simulink model "FCS"  (Simulink 9.1)
settings: Solver=VariableStepAuto  StartTime=0.0  StopTime=10.0  RelTol=1e-3
values from neighbouring files (symbols this model uses):
  Controller =     [data_set.mat]
  Estimator =     [data_set.mat]
  g = 9.81    [data_set.mat]
  init =     [data_set.mat]
  Sensors =     [data_set.mat]
  Ts = 0.005    [data_set.mat]
  Vehicle =     [data_set.mat]
undefined symbols (not defined in the file or in its folder): DiscIntNeverNeededParam, Discrete, Time
libraries: F_Line_block x470, simulink x33, ctrlSharedLib x3, sharedtransform x3, sharedutil x1
(part 1 of 3)
settings Model: LogicAnalyzerSignalOrdering=db974c0d-bb14-49c7-94ac-ee659e6fa1a8,d1d32620-0112-4d85-a8d5-fcd62d13050a  Creator=dongw  LastModifiedBy=dongw
settings DataIOCC: SaveFormat=Dataset
settings OptimizationCC: LifeSpan=auto
settings DebuggingCC: UnderspecifiedInitializationDetection=Simplified  MergeDetectMultiDrivingBlocksExec=error  SFUnexpectedBacktrackingDiag=error  SFNoUnconditionalDefaultTransitionDiag=error  SFExecutionAtInitializationDiag=warning
settings HardwareCC: ProdBitPerPointer=64  ProdBitPerSizeT=64  ProdBitPerPtrDiffT=64  ProdLargestAtomicFloat=Float  ProdIntDivRoundTo=Zero  ProdEndianess=LittleEndian  ProdWordSize=64  ProdHWDeviceType=Intel->x86-64 (Windows64)
settings ModelReferenceCC: PropagateSignalLabelsOutOfModel=on
settings CodeAppCC: StateflowObjectComments=off
settings GRTTargetCC: TargetLangStandard=C99 (ISO)  CombineOutputUpdateFcns=on  GRTInterface=off
settings ConfigComp: CovMetricSettings=dwe  CovHtmlReporting=off  CovSaveCumulativeToWorkspaceVar=off  CovSaveSingleToWorkspaceVar=off  CovExternalEMLEnable=on

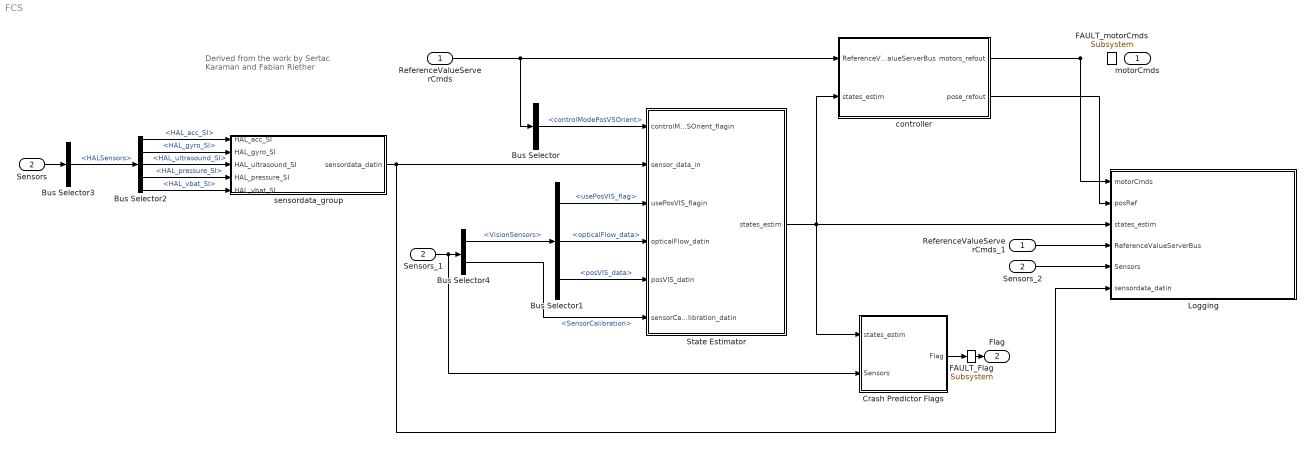
== system FCS ==
  note: Derived from the work by Sertac
      | Karaman and Fabian Riether
  ReferenceValueServerCmds : Inport  OutDataTypeStr=Bus: CommandBus
  Sensors : Inport  Port=2  OutDataTypeStr=Bus: SensorsBus  BusOutputAsStruct=on
  Bus Selector : BusSelector  OutputSignals=controlModePosVSOrient
  Bus Selector1 : BusSelector  OutputSignals=usePosVIS_flag,opticalFlow_data,posVIS_data
  Bus Selector2 : BusSelector  OutputSignals=HAL_acc_SI,HAL_gyro_SI,HAL_ultrasound_SI,HAL_pressure_SI,HAL_vbat_SI
  Bus Selector3 : BusSelector  OutputSignals=HALSensors
  Bus Selector4 : BusSelector  OutputSignals=VisionSensors,SensorCalibration
  Crash Predictor Flags : Subsystem
  Logging : Subsystem  TreatAsAtomicUnit=on
      settings: RTWFcnNameOpts=Use subsystem name
  ReferenceValueServerCmds_1 : InportShadow  OutDataTypeStr=Bus: CommandBus
  Sensors_1 : InportShadow  Port=2  OutDataTypeStr=Bus: SensorsBus  BusOutputAsStruct=on
  Sensors_2 : InportShadow  Port=2  OutDataTypeStr=Bus: SensorsBus  BusOutputAsStruct=on
  State Estimator : Subsystem
  controller : Subsystem
  sensordata_group : Subsystem
  motorCmds : Outport
  FAULT_motorCmds : F_Line_block/Subsystem
  Flag : Outport  Port=2
  FAULT_Flag : F_Line_block/Subsystem
  wires:
  sensordata_group/1(sensordata_datin) -> State Estimator/2(sensor_data_in), Logging/6(sensordata_datin)
  Bus Selector1/2 -> State Estimator/4(opticalFlow_datin)  "<opticalFlow_data>"
  Sensors_1/1 -> Crash Predictor Flags/2(Sensors), Bus Selector4/1
  Bus Selector2/3 -> sensordata_group/3(HAL_ultrasound_SI)  "<HAL_ultrasound_SI>"
  Bus Selector/1 -> State Estimator/1(controlModePosVSOrient_flagin)  "<controlModePosVSOrient>"
  Sensors/1 -> Bus Selector3/1
  Sensors_2/1 -> Logging/5(Sensors)
  Bus Selector2/2 -> sensordata_group/2(HAL_gyro_SI)  "<HAL_gyro_SI>"
  Bus Selector4/2 -> State Estimator/6(sensorCalibration_datin)  "<SensorCalibration>"
  Crash Predictor Flags/1(Flag) -> FAULT_Flag/1
  ?FAULT_Sum4_		DstPort			1/1 -> ?Sum4/dstport			1
  ?FAULT_Mux2_3/1 -> ?Mux2/3
  ?FAULT_pitch_roll_cmd/1 -> ?pitch_roll_cmd/1
  ?FAULT_Out Bus Element7/1 -> ?Out Bus Element7/1
  ?FAULT_Delay1/1 -> ?Delay1/1
  ?FAULT_Demux3/1 -> ?Demux3/1
  FAULT_Flag/1 -> Flag/1
  controller/1(motors_refout) -> ?FAULT_motorCmds_	DstPort			1/1, Logging/1(motorCmds)
  ?FAULT_motorCmds_	DstPort			1/1 -> motorCmds/dstport			1
  ?FAULT_Mux2_3/1 -> ?Mux2/3
  Bus Selector1/1 -> State Estimator/3(usePosVIS_flagin)  "<usePosVIS_flag>"
  Bus Selector1/3 -> State Estimator/5(posVIS_datin)  "<posVIS_data>"
  Bus Selector2/1 -> sensordata_group/1(HAL_acc_SI)  "<HAL_acc_SI>"
  controller/2(pose_refout) -> Logging/2(posRef)
  ReferenceValueServerCmds_1/1 -> Logging/4(ReferenceValueServerBus)
  Bus Selector4/1 -> Bus Selector1/1  "<VisionSensors>"
  State Estimator/1(states_estim) -> controller/2(states_estim), Crash Predictor Flags/1(states_estim), Logging/3(states_estim)
  Bus Selector2/5 -> sensordata_group/5(HAL_vbat_SI)  "<HAL_vbat_SI>"
  Bus Selector2/4 -> sensordata_group/4(HAL_pressure_SI)  "<HAL_pressure_SI>"
  Bus Selector3/1 -> Bus Selector2/1  "<HALSensors>"
  ReferenceValueServerCmds/1 -> controller/1(ReferenceValueServerBus), Bus Selector/1

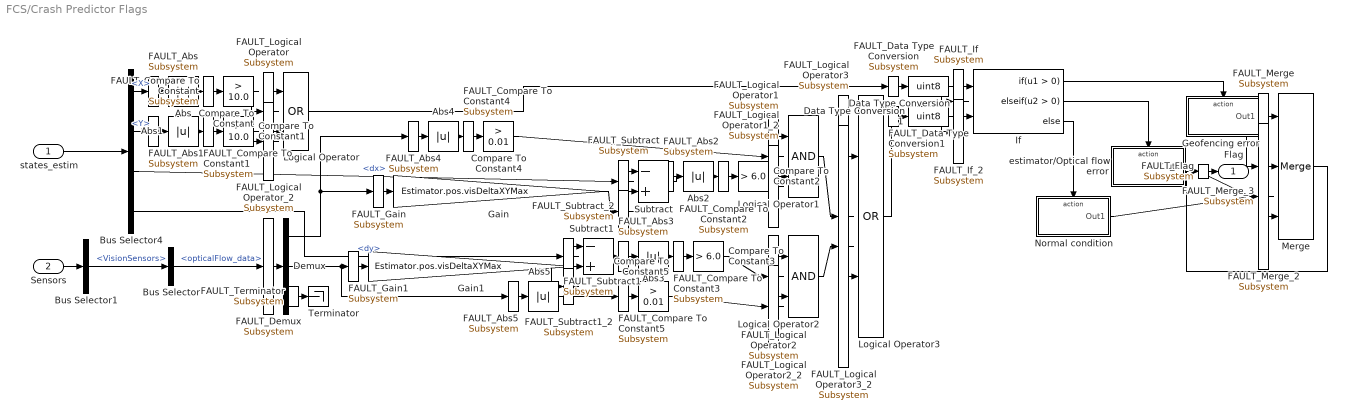
== system FCS/Crash Predictor Flags ==
  states_estim : Inport
  Sensors : Inport  Port=2
  Abs{,1..5} (6 alike) : Abs
  FAULT_Abs{,1..5} (6 alike) : F_Line_block/Subsystem
  Bus Selector : BusSelector  OutputSignals=opticalFlow_data
  Bus Selector1 : BusSelector  OutputSignals=VisionSensors
  Bus Selector4 : BusSelector  OutputSignals=X,Y,dx,dy
  Compare To Constant : simulink/Logic and Bit Operations/Compare To Constant  relop=>  const=10.0  OutDataTypeStr=boolean
  FAULT_Compare To Constant{,1..5} (6 alike) : F_Line_block/Subsystem
  Compare To Constant1 : simulink/Logic and Bit Operations/Compare To Constant  relop=>  const=10.0  OutDataTypeStr=boolean
  Compare To Constant2 : simulink/Logic and Bit Operations/Compare To Constant  relop=>  const=6.0  OutDataTypeStr=boolean
  Compare To Constant3 : simulink/Logic and Bit Operations/Compare To Constant  relop=>  const=6.0  OutDataTypeStr=boolean
  Compare To Constant4 : simulink/Logic and Bit Operations/Compare To Constant  relop=>  const=0.01  OutDataTypeStr=boolean
  Compare To Constant5 : simulink/Logic and Bit Operations/Compare To Constant  relop=>  const=0.01  OutDataTypeStr=boolean
  Data Type Conversion : DataTypeConversion  OutDataTypeStr=uint8  RndMeth=Nearest
  FAULT_Data Type Conversion : F_Line_block/Subsystem
  Data Type Conversion1 : DataTypeConversion  OutDataTypeStr=uint8  RndMeth=Nearest
  FAULT_Data Type Conversion1 : F_Line_block/Subsystem
  Demux : Demux  Outputs=3
  FAULT_Demux : F_Line_block/Subsystem
  Gain : Gain  Gain=Estimator.pos.visDeltaXYMax
  FAULT_Gain : F_Line_block/Subsystem
  Gain1 : Gain  Gain=Estimator.pos.visDeltaXYMax
  FAULT_Gain1 : F_Line_block/Subsystem
  Geofencing error : Subsystem  TreatAsAtomicUnit=on
  If : If  NumInputs=2  ElseIfExpressions=u2 > 0
  FAULT_If : F_Line_block/Subsystem
  FAULT_If_2 : F_Line_block/Subsystem
  Logical Operator : Logic  Operator=OR  AllPortsSameDT=off
  FAULT_Logical Operator{,1..3} (4 alike) : F_Line_block/Subsystem
  FAULT_Logical Operator_2 : F_Line_block/Subsystem
  Logical Operator1 : Logic  AllPortsSameDT=off  OutDataTypeStr=boolean
  FAULT_Logical Operator1_2 : F_Line_block/Subsystem
  Logical Operator2 : Logic  AllPortsSameDT=off  OutDataTypeStr=boolean
  FAULT_Logical Operator2_2 : F_Line_block/Subsystem
  Logical Operator3 : Logic  Operator=OR  AllPortsSameDT=off
  FAULT_Logical Operator3_2 : F_Line_block/Subsystem
  Merge : Merge  Inputs=3  InitialOutput=0
  FAULT_Merge : F_Line_block/Subsystem
  FAULT_Merge_2 : F_Line_block/Subsystem
  FAULT_Merge_3 : F_Line_block/Subsystem
  Normal condition : Subsystem  TreatAsAtomicUnit=on
  Subtract : Sum  Inputs=-+
  FAULT_Subtract : F_Line_block/Subsystem
  FAULT_Subtract_2 : F_Line_block/Subsystem
  Subtract1 : Sum  Inputs=-+
  FAULT_Subtract1 : F_Line_block/Subsystem
  FAULT_Subtract1_2 : F_Line_block/Subsystem
  Terminator : Terminator
  FAULT_Terminator : F_Line_block/Subsystem
  estimator/Optical flow error : Subsystem  TreatAsAtomicUnit=on
  Flag : Outport
  FAULT_Flag : F_Line_block/Subsystem
  wires:
  Bus Selector4/1 -> FAULT_Abs/1  "<X>"
  FAULT_Abs/1 -> Abs/1
  states_estim/1 -> Bus Selector4/1
  Bus Selector4/2 -> FAULT_Abs1/1  "<Y>"
  FAULT_Abs1/1 -> Abs1/1
  Compare To Constant/1 -> FAULT_Logical Operator/1
  FAULT_Logical Operator/1 -> Logical Operator/1
  Compare To Constant1/1 -> FAULT_Logical Operator_2/1
  FAULT_Logical Operator_2/1 -> Logical Operator/2
  Abs/1 -> FAULT_Compare To Constant/1
  FAULT_Compare To Constant/1 -> Compare To Constant/1
  Abs1/1 -> FAULT_Compare To Constant1/1
  FAULT_Compare To Constant1/1 -> Compare To Constant1/1
  Logical Operator/1 -> FAULT_Data Type Conversion/1
  FAULT_Data Type Conversion/1 -> Data Type Conversion/1
  Bus Selector/1 -> FAULT_Demux/1  "<opticalFlow_data>"
  FAULT_Demux/1 -> Demux/1
  Demux/1 -> FAULT_Abs4/1, FAULT_Gain/1
  FAULT_Abs4/1 -> Abs4/1
  FAULT_Gain/1 -> Gain/1
  Demux/2 -> FAULT_Gain1/1, FAULT_Abs5/1
  FAULT_Gain1/1 -> Gain1/1
  FAULT_Abs5/1 -> Abs5/1
  Bus Selector4/3 -> FAULT_Subtract/1  "<dx>"
  FAULT_Subtract/1 -> Subtract/1
  Subtract/1 -> FAULT_Abs2/1
  FAULT_Abs2/1 -> Abs2/1
  Subtract1/1 -> FAULT_Abs3/1
  FAULT_Abs3/1 -> Abs3/1
  Abs2/1 -> FAULT_Compare To Constant2/1
  FAULT_Compare To Constant2/1 -> Compare To Constant2/1
  Abs3/1 -> FAULT_Compare To Constant3/1
  FAULT_Compare To Constant3/1 -> Compare To Constant3/1
  Compare To Constant5/1 -> FAULT_Logical Operator2_2/1
  FAULT_Logical Operator2_2/1 -> Logical Operator2/2
  Abs4/1 -> FAULT_Compare To Constant4/1
  FAULT_Compare To Constant4/1 -> Compare To Constant4/1
  Abs5/1 -> FAULT_Compare To Constant5/1
  FAULT_Compare To Constant5/1 -> Compare To Constant5/1
  Compare To Constant3/1 -> FAULT_Logical Operator2/1
  FAULT_Logical Operator2/1 -> Logical Operator2/1
  Logical Operator1/1 -> FAULT_Logical Operator3/1
  FAULT_Logical Operator3/1 -> Logical Operator3/1
  Logical Operator2/1 -> FAULT_Logical Operator3_2/1
  FAULT_Logical Operator3_2/1 -> Logical Operator3/2
  Logical Operator3/1 -> FAULT_Data Type Conversion1/1
  FAULT_Data Type Conversion1/1 -> Data Type Conversion1/1
  Demux/3 -> FAULT_Terminator/1
  FAULT_Terminator/1 -> Terminator/1
  Gain/1 -> FAULT_Subtract_2/1
  FAULT_Subtract_2/1 -> Subtract/2
  Bus Selector4/4 -> FAULT_Subtract1/1  "<dy>"
  FAULT_Subtract1/1 -> Subtract1/1
  Gain1/1 -> FAULT_Subtract1_2/1
  FAULT_Subtract1_2/1 -> Subtract1/2
  Compare To Constant4/1 -> FAULT_Logical Operator1/1
  FAULT_Logical Operator1/1 -> Logical Operator1/1
  Compare To Constant2/1 -> FAULT_Logical Operator1_2/1
  FAULT_Logical Operator1_2/1 -> Logical Operator1/2
  Sensors/1 -> Bus Selector1/1
  Bus Selector1/1 -> Bus Selector/1  "<VisionSensors>"
  Merge/1 -> FAULT_Flag/1
  FAULT_Flag/1 -> Flag/1
  If/1 -> Geofencing error/Action
  If/2 -> estimator/Optical flow error/Action
  If/3 -> Normal condition/Action
  Geofencing error/1(Out1) -> FAULT_Merge/1
  FAULT_Merge/1 -> Merge/1
  estimator/Optical flow error/1(Out1) -> FAULT_Merge_2/1
  FAULT_Merge_2/1 -> Merge/2
  Normal condition/1(Out1) -> FAULT_Merge_3/1
  FAULT_Merge_3/1 -> Merge/3
  Data Type Conversion/1 -> FAULT_If/1
  FAULT_If/1 -> If/1
  Data Type Conversion1/1 -> FAULT_If_2/1
  FAULT_If_2/1 -> If/2

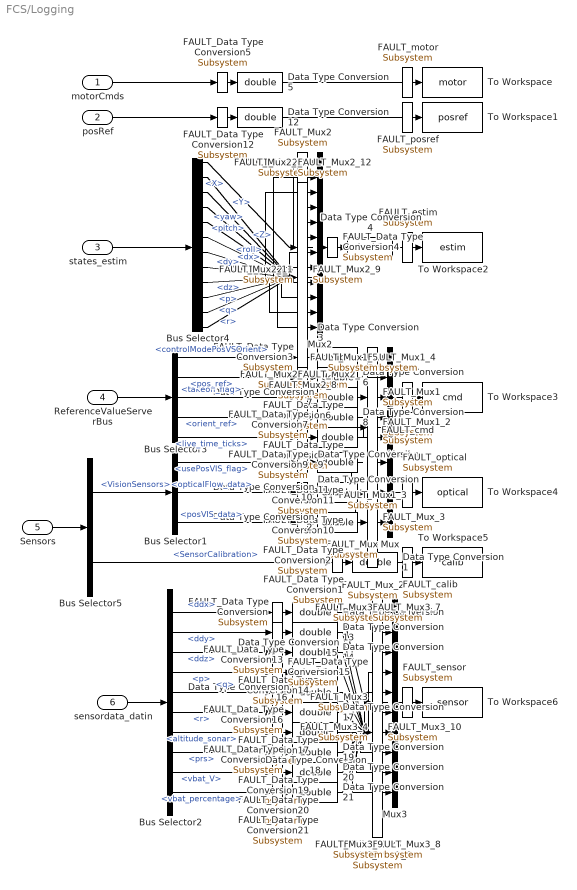
== system FCS/Logging ==
  motorCmds : Inport
  posRef : Inport  Port=2
  states_estim : Inport  Port=3  OutDataTypeStr=Bus: statesEstim_t  BusOutputAsStruct=on
  ReferenceValueServerBus : Inport  Port=4  OutDataTypeStr=Bus: CommandBus  BusOutputAsStruct=on
  Sensors : Inport  Port=5  OutDataTypeStr=Bus: SensorsBus
  sensordata_datin : Inport  Port=6  OutDataTypeStr=Bus: sensordata_t
  Bus Selector1 : BusSelector  OutputSignals=usePosVIS_flag,opticalFlow_data,posVIS_data
  Bus Selector2 : BusSelector  OutputSignals=ddx,ddy,ddz,p,q,r,altitude_sonar,prs,vbat_V,vbat_percentage
  Bus Selector3 : BusSelector  OutputSignals=controlModePosVSOrient,pos_ref,takeoff_flag,orient_ref,live_time_ticks
  Bus Selector4 : BusSelector  OutputSignals=X,Y,Z,yaw,pitch,roll,dx,dy,dz,p,q,r
  Bus Selector5 : BusSelector  OutputSignals=VisionSensors,SensorCalibration
  Data Type Conversion{,1..21} (22 alike) : DataTypeConversion  OutDataTypeStr=double
  FAULT_Data Type Conversion{,1..21} (22 alike) : F_Line_block/Subsystem
  Mux : Mux  Inputs=3
  FAULT_Mux{,1..3} (4 alike) : F_Line_block/Subsystem
  FAULT_Mux_2 : F_Line_block/Subsystem
  FAULT_Mux_3 : F_Line_block/Subsystem
  Mux1 : Mux  Inputs=5
  FAULT_Mux1_{2..5} (4 alike) : F_Line_block/Subsystem
  Mux2 : Mux  Inputs=12
  FAULT_Mux2_{2..12} (11 alike) : F_Line_block/Subsystem
  Mux3 : Mux  Inputs=10
  FAULT_Mux3_{2..10} (9 alike) : F_Line_block/Subsystem
  To Workspace : ToWorkspace  VariableName=motor  SaveFormat=Structure With Time  SampleTime=-1
  FAULT_motor : F_Line_block/Subsystem
  To Workspace1 : ToWorkspace  VariableName=posref  SaveFormat=Structure With Time  SampleTime=-1
  FAULT_posref : F_Line_block/Subsystem
  To Workspace2 : ToWorkspace  VariableName=estim  SaveFormat=Structure With Time  SampleTime=-1
  FAULT_estim : F_Line_block/Subsystem
  To Workspace3 : ToWorkspace  VariableName=cmd  SaveFormat=Structure With Time  SampleTime=-1
  FAULT_cmd : F_Line_block/Subsystem
  To Workspace4 : ToWorkspace  VariableName=optical  SaveFormat=Structure With Time  SampleTime=-1
  FAULT_optical : F_Line_block/Subsystem
  To Workspace5 : ToWorkspace  VariableName=calib  SaveFormat=Structure With Time  SampleTime=-1
  FAULT_calib : F_Line_block/Subsystem
  To Workspace6 : ToWorkspace  VariableName=sensor  SaveFormat=Structure With Time  SampleTime=-1
  FAULT_sensor : F_Line_block/Subsystem
  wires:
  Bus Selector3/1 -> FAULT_Data Type Conversion3/1  "<controlModePosVSOrient>"
  FAULT_Data Type Conversion3/1 -> Data Type Conversion3/1
  Bus Selector3/3 -> FAULT_Data Type Conversion7/1  "<takeoff_flag>"
  FAULT_Data Type Conversion7/1 -> Data Type Conversion7/1
  Bus Selector3/4 -> FAULT_Data Type Conversion8/1  "<orient_ref>"
  FAULT_Data Type Conversion8/1 -> Data Type Conversion8/1
  Bus Selector3/5 -> FAULT_Data Type Conversion9/1  "<live_time_ticks>"
  FAULT_Data Type Conversion9/1 -> Data Type Conversion9/1
  ReferenceValueServerBus/1 -> Bus Selector3/1
  Bus Selector3/2 -> FAULT_Data Type Conversion6/1  "<pos_ref>"
  FAULT_Data Type Conversion6/1 -> Data Type Conversion6/1
  sensordata_datin/1 -> Bus Selector2/1
  Bus Selector2/1 -> FAULT_Data Type Conversion/1  "<ddx>"
  FAULT_Data Type Conversion/1 -> Data Type Conversion/1
  Sensors/1 -> Bus Selector5/1
  Bus Selector1/1 -> FAULT_Data Type Conversion11/1  "<usePosVIS_flag>"
  FAULT_Data Type Conversion11/1 -> Data Type Conversion11/1
  Bus Selector1/2 -> FAULT_Data Type Conversion10/1  "<opticalFlow_data>"
  FAULT_Data Type Conversion10/1 -> Data Type Conversion10/1
  Bus Selector1/3 -> FAULT_Data Type Conversion2/1  "<posVIS_data>"
  FAULT_Data Type Conversion2/1 -> Data Type Conversion2/1
  Data Type Conversion1/1 -> To Workspace5/1
  Bus Selector5/2 -> FAULT_Data Type Conversion1/1  "<SensorCalibration>"
  FAULT_Data Type Conversion1/1 -> Data Type Conversion1/1
  Mux/1 -> To Workspace4/1
  Data Type Conversion4/1 -> To Workspace2/1
  motorCmds/1 -> FAULT_Data Type Conversion5/1
  FAULT_Data Type Conversion5/1 -> Data Type Conversion5/1
  Data Type Conversion5/1 -> To Workspace/1
  Mux1/1 -> To Workspace3/1
  states_estim/1 -> Bus Selector4/1
  Mux2/1 -> FAULT_Data Type Conversion4/1
  FAULT_Data Type Conversion4/1 -> Data Type Conversion4/1
  Bus Selector4/4 -> FAULT_Mux2_4/1  "<yaw>"
  FAULT_Mux2_4/1 -> Mux2/4
  Bus Selector4/6 -> FAULT_Mux2_6/1  "<roll>"
  FAULT_Mux2_6/1 -> Mux2/6
  Bus Selector4/5 -> FAULT_Mux2_5/1  "<pitch>"
  FAULT_Mux2_5/1 -> Mux2/5
  Bus Selector4/9 -> FAULT_Mux2_9/1  "<dz>"
  FAULT_Mux2_9/1 -> Mux2/9
  Bus Selector4/7 -> FAULT_Mux2_7/1  "<dx>"
  FAULT_Mux2_7/1 -> Mux2/7
  Bus Selector4/8 -> FAULT_Mux2_8/1  "<dy>"
  FAULT_Mux2_8/1 -> Mux2/8
  Bus Selector4/10 -> FAULT_Mux2_10/1  "<p>"
  FAULT_Mux2_10/1 -> Mux2/10
  Bus Selector4/12 -> FAULT_Mux2_12/1  "<r>"
  FAULT_Mux2_12/1 -> Mux2/12
  Bus Selector4/2 -> FAULT_Mux2_2/1  "<Y>"
  FAULT_Mux2_2/1 -> Mux2/2
  Bus Selector4/11 -> FAULT_Mux2_11/1  "<q>"
  FAULT_Mux2_11/1 -> Mux2/11
  Bus Selector4/3 -> FAULT_Mux2_3/1  "<Z>"
  FAULT_Mux2_3/1 -> Mux2/3
  Bus Selector4/1 -> FAULT_Mux2/1  "<X>"
  FAULT_Mux2/1 -> Mux2/1
  Data Type Conversion3/1 -> FAULT_Mux1/1
  FAULT_Mux1/1 -> Mux1/1
  Data Type Conversion6/1 -> FAULT_Mux1_2/1
  FAULT_Mux1_2/1 -> Mux1/2
  Data Type Conversion7/1 -> FAULT_Mux1_3/1
  FAULT_Mux1_3/1 -> Mux1/3
  Data Type Conversion8/1 -> FAULT_Mux1_4/1
  FAULT_Mux1_4/1 -> Mux1/4
  Data Type Conversion9/1 -> FAULT_Mux1_5/1
  FAULT_Mux1_5/1 -> Mux1/5
  Data Type Conversion2/1 -> FAULT_Mux_3/1
  FAULT_Mux_3/1 -> Mux/3
  Data Type Conversion10/1 -> FAULT_Mux_2/1
  FAULT_Mux_2/1 -> Mux/2
  Data Type Conversion11/1 -> FAULT_Mux/1
  FAULT_Mux/1 -> Mux/1
  posRef/1 -> FAULT_Data Type Conversion12/1
  FAULT_Data Type Conversion12/1 -> Data Type Conversion12/1
  Data Type Conversion12/1 -> To Workspace1/1
  Bus Selector2/2 -> FAULT_Data Type Conversion13/1  "<ddy>"
  FAULT_Data Type Conversion13/1 -> Data Type Conversion13/1
  Bus Selector2/3 -> FAULT_Data Type Conversion14/1  "<ddz>"
  FAULT_Data Type Conversion14/1 -> Data Type Conversion14/1
  Bus Selector2/4 -> FAULT_Data Type Conversion15/1  "<p>"
  FAULT_Data Type Conversion15/1 -> Data Type Conversion15/1
  Bus Selector2/5 -> FAULT_Data Type Conversion16/1  "<q>"
  FAULT_Data Type Conversion16/1 -> Data Type Conversion16/1
  Bus Selector2/6 -> FAULT_Data Type Conversion17/1  "<r>"
  FAULT_Data Type Conversion17/1 -> Data Type Conversion17/1
  Bus Selector2/7 -> FAULT_Data Type Conversion18/1  "<altitude_sonar>"
  FAULT_Data Type Conversion18/1 -> Data Type Conversion18/1
  Bus Selector2/8 -> FAULT_Data Type Conversion19/1  "<prs>"
  FAULT_Data Type Conversion19/1 -> Data Type Conversion19/1
  Bus Selector2/9 -> FAULT_Data Type Conversion20/1  "<vbat_V>"
  FAULT_Data Type Conversion20/1 -> Data Type Conversion20/1
  Bus Selector2/10 -> FAULT_Data Type Conversion21/1  "<vbat_percentage>"
  FAULT_Data Type Conversion21/1 -> Data Type Conversion21/1
  Data Type Conversion/1 -> FAULT_Mux3/1
  FAULT_Mux3/1 -> Mux3/1
  Data Type Conversion13/1 -> FAULT_Mux3_2/1
  FAULT_Mux3_2/1 -> Mux3/2
  Data Type Conversion14/1 -> FAULT_Mux3_3/1
  FAULT_Mux3_3/1 -> Mux3/3
  Data Type Conversion15/1 -> FAULT_Mux3_4/1
  FAULT_Mux3_4/1 -> Mux3/4
  Data Type Conversion16/1 -> FAULT_Mux3_5/1
  FAULT_Mux3_5/1 -> Mux3/5
  Data Type Conversion17/1 -> FAULT_Mux3_6/1
  FAULT_Mux3_6/1 -> Mux3/6
  Data Type Conversion18/1 -> FAULT_Mux3_7/1
  FAULT_Mux3_7/1 -> Mux3/7
  Data Type Conversion19/1 -> FAULT_Mux3_8/1
  FAULT_Mux3_8/1 -> Mux3/8
  Data Type Conversion20/1 -> FAULT_Mux3_9/1
  FAULT_Mux3_9/1 -> Mux3/9
  Data Type Conversion21/1 -> FAULT_Mux3_10/1
  FAULT_Mux3_10/1 -> Mux3/10
  Mux3/1 -> To Workspace6/1
  Bus Selector5/1 -> Bus Selector1/1  "<VisionSensors>"

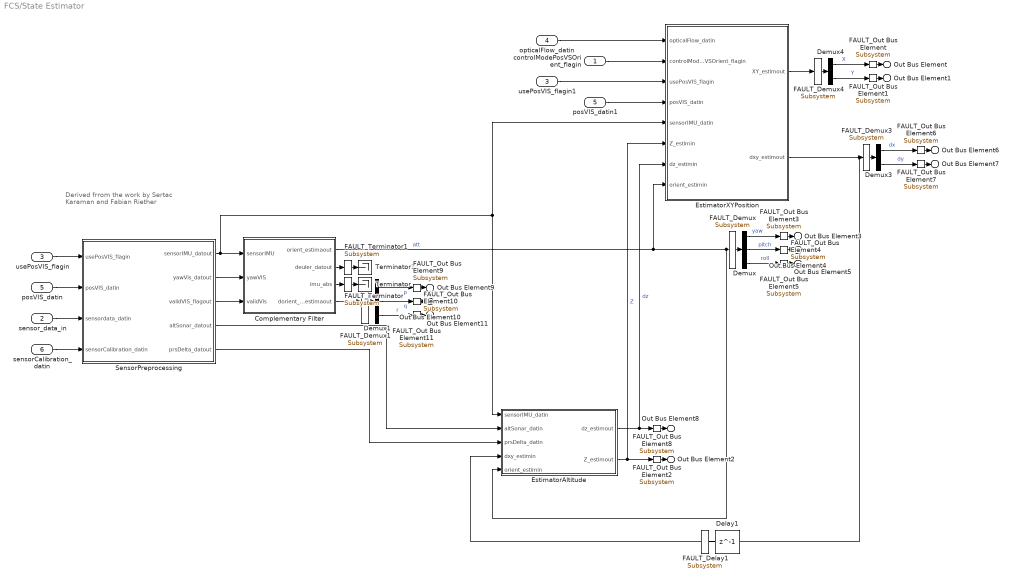
== system FCS/State Estimator ==
  note: Derived frrom the work by Sertac
      | Karaman and Fabian Riether
  controlModePosVSOrient_flagin : Inport  OutDataTypeStr=boolean
  sensor_data_in : Inport  Port=2
  usePosVIS_flagin : Inport  Port=3
  opticalFlow_datin : Inport  Port=4
  posVIS_datin : Inport  Port=5
  sensorCalibration_datin : Inport  Port=6
  Complementary Filter : Subsystem
  Delay1 : Delay  DelayLength=1  InitialCondition=0
  FAULT_Delay1 : F_Line_block/Subsystem
  Demux : Demux  Outputs=3
  FAULT_Demux{,1,3..4} (4 alike) : F_Line_block/Subsystem
  Demux1 : Demux  Outputs=3
  Demux3 : Demux  Outputs=2
  Demux4 : Demux  Outputs=2
  EstimatorAltitude : Subsystem
  EstimatorXYPosition : Subsystem
  SensorPreprocessing : Subsystem
  Terminator : Terminator
  FAULT_Terminator : F_Line_block/Subsystem
  Terminator1 : Terminator
  FAULT_Terminator1 : F_Line_block/Subsystem
  posVIS_datin1 : InportShadow  Port=5
  usePosVIS_flagin1 : InportShadow  Port=3
  Out Bus Element : Outport  PortName=states_estim  Element=X
  FAULT_Out Bus Element{,1..11} (12 alike) : F_Line_block/Subsystem
  Out Bus Element1 : Outport  PortName=states_estim  Element=Y
  Out Bus Element2 : Outport  PortName=states_estim  Element=Z
  Out Bus Element3 : Outport  PortName=states_estim  Element=yaw
  Out Bus Element4 : Outport  PortName=states_estim  Element=pitch
  Out Bus Element5 : Outport  PortName=states_estim  Element=roll
  Out Bus Element6 : Outport  PortName=states_estim  Element=dx
  Out Bus Element7 : Outport  PortName=states_estim  Element=dy
  Out Bus Element8 : Outport  PortName=states_estim  Element=dz
  Out Bus Element9 : Outport  PortName=states_estim  Element=p
  Out Bus Element10 : Outport  PortName=states_estim  Element=q
  Out Bus Element11 : Outport  PortName=states_estim  Element=r
  wires:
  EstimatorXYPosition/2(dxy_estimout) -> FAULT_Delay1/1, FAULT_Demux3/1
  ?FAULT_dxy_estimout_		DstPort			1/1 -> ?dxy_estimout/dstport			1
  ?FAULT_KalmanFilter_posxy/1 -> ?KalmanFilter_posxy/1
  ?FAULT_Mux1_6/1 -> ?Mux1/6
  ?FAULT_Product_2/1 -> ?Product/2
  FAULT_Delay1/1 -> Delay1/1
  FAULT_Demux3/1 -> Demux3/1
  posVIS_datin/1 -> SensorPreprocessing/2(posVIS_datin)
  Demux1/3 -> FAULT_Out Bus Element11/1  "r"
  FAULT_Out Bus Element11/1 -> Out Bus Element11/1
  Demux/3 -> FAULT_Out Bus Element5/1  "roll"
  FAULT_Out Bus Element5/1 -> Out Bus Element5/1
  Demux4/2 -> FAULT_Out Bus Element1/1  "Y"
  FAULT_Out Bus Element1/1 -> Out Bus Element1/1
  EstimatorXYPosition/1(XY_estimout) -> FAULT_Demux4/1
  FAULT_Demux4/1 -> Demux4/1
  Complementary Filter/2(deuler_datout) -> FAULT_Terminator1/1
  FAULT_Terminator1/1 -> Terminator1/1
  Complementary Filter/4(dorient_estimaout) -> FAULT_Demux1/1
  FAULT_Demux1/1 -> Demux1/1
  SensorPreprocessing/3(validVIS_flagout) -> Complementary Filter/3(validVis)
  sensor_data_in/1 -> SensorPreprocessing/3(sensordata_datin)
  opticalFlow_datin/1 -> EstimatorXYPosition/1(opticalFlow_datin)
  Demux4/1 -> FAULT_Out Bus Element/1  "X"
  FAULT_Out Bus Element/1 -> Out Bus Element/1
  SensorPreprocessing/1(sensorIMU_datout) -> Complementary Filter/1(sensorIMU), EstimatorAltitude/1(sensorIMU_datin), EstimatorXYPosition/5(sensorIMU_datin)
  SensorPreprocessing/5(prsDelta_datout) -> EstimatorAltitude/3(prsDelta_datin)
  Demux3/2 -> FAULT_Out Bus Element7/1  "dy"
  ?FAULT_dxy_estimout_		DstPort			1/1 -> ?dxy_estimout/dstport			1
  ?FAULT_KalmanFilter_posxy/1 -> ?KalmanFilter_posxy/1
  ?FAULT_Mux1_6/1 -> ?Mux1/6
  FAULT_Out Bus Element7/1 -> Out Bus Element7/1
  SensorPreprocessing/2(yawVis_datout) -> Complementary Filter/2(yawVIS)
  SensorPreprocessing/4(altSonar_datout) -> EstimatorAltitude/2(altSonar_datin)
  usePosVIS_flagin/1 -> SensorPreprocessing/1(usePosVIS_flagin)
  EstimatorAltitude/1(dz_estimout) -> FAULT_Out Bus Element8/1, EstimatorXYPosition/7(dz_estimin)  "dz"
  FAULT_Out Bus Element8/1 -> Out Bus Element8/1
  ?FAULT_KalmanFilter_posxy/1 -> ?KalmanFilter_posxy/1
  EstimatorAltitude/2(Z_estimout) -> FAULT_Out Bus Element2/1, EstimatorXYPosition/6(Z_estimin)  "Z"
  FAULT_Out Bus Element2/1 -> Out Bus Element2/1
  ?FAULT_KalmanFilter_posxy/1 -> ?KalmanFilter_posxy/1
  Demux1/1 -> FAULT_Out Bus Element9/1  "p"
  FAULT_Out Bus Element9/1 -> Out Bus Element9/1
  Demux3/1 -> FAULT_Out Bus Element6/1  "dx"
  FAULT_Out Bus Element6/1 -> Out Bus Element6/1
  Complementary Filter/3(imu_abs) -> FAULT_Terminator/1
  FAULT_Terminator/1 -> Terminator/1
  Demux/2 -> FAULT_Out Bus Element4/1  "pitch"
  FAULT_Out Bus Element4/1 -> Out Bus Element4/1
  controlModePosVSOrient_flagin/1 -> EstimatorXYPosition/2(controlModePosVSOrient_flagin)
  Complementary Filter/1(orient_estimaout) -> EstimatorAltitude/5(orient_estimin), Demux/1, EstimatorXYPosition/8(orient_estimin)  "att"
  Demux/1 -> FAULT_Out Bus Element3/1  "yaw"
  FAULT_Out Bus Element2/1 -> Out Bus Element2/1
  FAULT_Out Bus Element3/1 -> Out Bus Element3/1
  Delay1/1 -> EstimatorAltitude/4(dxy_estimin)
  Demux1/2 -> FAULT_Out Bus Element10/1  "q"
  FAULT_Out Bus Element10/1 -> Out Bus Element10/1
  usePosVIS_flagin1/1 -> EstimatorXYPosition/3(usePosVIS_flagin)
  posVIS_datin1/1 -> EstimatorXYPosition/4(posVIS_datin)
  sensorCalibration_datin/1 -> SensorPreprocessing/4(sensorCalibration_datin)

== system FCS/controller ==
  In Bus Element1 : Inport  PortName=ReferenceValueServerBus  Element=controlModePosVSOrient
  In Bus Element : Inport  PortName=ReferenceValueServerBus  Element=pos_ref
  In Bus Element4 : Inport  PortName=ReferenceValueServerBus  Element=pos_ref
  In Bus Element5 : Inport  PortName=ReferenceValueServerBus  Element=pos_ref
  In Bus Element2 : Inport  PortName=ReferenceValueServerBus  Element=orient_ref
  In Bus Element6 : Inport  PortName=ReferenceValueServerBus  Element=orient_ref
  In Bus Element7 : Inport  PortName=ReferenceValueServerBus  Element=orient_ref
  In Bus Element3 : Inport  PortName=ReferenceValueServerBus  Element=takeoff_flag
  states_estim : Inport  Port=2
  Attitude : Subsystem
  ControlMixer : Subsystem
  Mux2 : Mux  Inputs=3
  FAULT_Mux2 : F_Line_block/Subsystem
  FAULT_Mux2_2 : F_Line_block/Subsystem
  FAULT_Mux2_3 : F_Line_block/Subsystem
  Selector : Selector  InputPortWidth=3  IndexOptions=Index vector (dialog)  Indices=3  OutputSizes=1
  Selector1 : Selector  InputPortWidth=3  IndexOptions=Index vector (dialog)  Indices=[1 2]  OutputSizes=1
  Selector2 : Selector  InputPortWidth=3  IndexOptions=Index vector (dialog)  Indices=[2 3]  OutputSizes=1
  Selector3 : Selector  InputPortWidth=3  IndexOptions=Index vector (dialog)  Indices=1  OutputSizes=1
  Switch_refAtt : Switch  Criteria=u2 > Threshold
  XY-to-reference-orientation : Subsystem
  Yaw : Subsystem
  gravity feedforward/equilibrium thrust : Subsystem
  states_estim1 : InportShadow  Port=2
  states_estim2 : InportShadow  Port=2
  states_estim3 : InportShadow  Port=2
  thrustsToMotorCommands : Subsystem
  motors_refout : Outport
  FAULT_motors_refout : F_Line_block/Subsystem
  pose_refout : Outport  Port=2
  FAULT_pose_refout : F_Line_block/Subsystem
  wires:
  thrustsToMotorCommands/1(motors_cmdout) -> FAULT_motors_refout/1
  FAULT_motors_refout/1 -> motors_refout/1
  In Bus Element1/1 -> Switch_refAtt/2
  XY-to-reference-orientation/1(pitch_roll_cmd) -> Switch_refAtt/1
  In Bus Element2/1 -> Selector3/1
  In Bus Element/1 -> Selector1/1
  Selector3/1 -> Yaw/1(yaw_ref)
  Selector1/1 -> XY-to-reference-orientation/1(posXY)  "pos"
  ControlMixer/1(thrusts_refout) -> thrustsToMotorCommands/1(thrusts_refin)
  In Bus Element3/1 -> gravity feedforward/equilibrium thrust/3(takeoff_flag)
  states_estim/1 -> Yaw/2(states_estim)
  Switch_refAtt/1 -> Attitude/1(refAttitude), FAULT_Mux2_3/1
  ?FAULT_Sum4_		DstPort			1/1 -> ?Sum4/dstport			1
  FAULT_Mux2_3/1 -> Mux2/3
  Yaw/1(yaw) -> XY-to-reference-orientation/3(yaw)
  gravity feedforward/equilibrium thrust/1(altitude_cmd) -> ControlMixer/4(totalThrust)
  Mux2/1 -> FAULT_pose_refout/1
  FAULT_pose_refout/1 -> pose_refout/1
  Attitude/1(tau_pitch) -> ControlMixer/1(tau_pitch)
  Attitude/2(tau_roll) -> ControlMixer/2(tau_roll)
  Yaw/2(tau_yaw) -> ControlMixer/3(tau_yaw)
  states_estim1/1 -> gravity feedforward/equilibrium thrust/1(states_estim)
  states_estim2/1 -> Attitude/2(states_estim)
  states_estim3/1 -> XY-to-reference-orientation/2(states_estim)
  In Bus Element4/1 -> FAULT_Mux2/1
  FAULT_Mux2/1 -> Mux2/1
  Selector/1 -> gravity feedforward/equilibrium thrust/2(PosZ)
  In Bus Element5/1 -> Selector/1
  In Bus Element6/1 -> Selector2/1
  Selector2/1 -> Switch_refAtt/3
  In Bus Element7/1 -> FAULT_Mux2_2/1
  FAULT_Mux2_2/1 -> Mux2/2

== system FCS/sensordata_group ==
  HAL_acc_SI : Inport  OutDataTypeStr=Bus: HAL_acc_SI_t
  HAL_gyro_SI : Inport  Port=2  OutDataTypeStr=Bus: HAL_gyro_SI_t
  HAL_ultrasound_SI : Inport  Port=3  OutDataTypeStr=Bus: HAL_ultrasound_SI_t
  HAL_pressure_SI : Inport  Port=4  OutDataTypeStr=Bus: HAL_pressure_SI_t
  HAL_vbat_SI : Inport  Port=5  OutDataTypeStr=Bus: HAL_vbat_SI_t
  Bus Selector1 : BusSelector  OutputSignals=vbat_V,vbat_percentage
  Bus Selector3 : BusSelector  OutputSignals=x,y,z
  Bus Selector4 : BusSelector  OutputSignals=x,y,z
  Bus Selector5 : BusSelector  OutputSignals=altitude
  Bus Selector6 : BusSelector  OutputSignals=pressure
  Out Bus Element : Outport  PortName=sensordata_datin  Element=ddx
  FAULT_Out Bus Element{,1..9} (10 alike) : F_Line_block/Subsystem
  Out Bus Element1 : Outport  PortName=sensordata_datin  Element=ddy
  Out Bus Element2 : Outport  PortName=sensordata_datin  Element=ddz
  Out Bus Element3 : Outport  PortName=sensordata_datin  Element=p
  Out Bus Element4 : Outport  PortName=sensordata_datin  Element=q
  Out Bus Element5 : Outport  PortName=sensordata_datin  Element=r
  Out Bus Element6 : Outport  PortName=sensordata_datin  Element=altitude_sonar
  Out Bus Element7 : Outport  PortName=sensordata_datin  Element=prs
  Out Bus Element8 : Outport  PortName=sensordata_datin  Element=vbat_V
  Out Bus Element9 : Outport  PortName=sensordata_datin  Element=vbat_percentage
  wires:
  HAL_gyro_SI/1 -> Bus Selector4/1
  HAL_acc_SI/1 -> Bus Selector3/1
  HAL_pressure_SI/1 -> Bus Selector6/1
  HAL_ultrasound_SI/1 -> Bus Selector5/1
  Bus Selector4/1 -> FAULT_Out Bus Element3/1  "<x>"
  FAULT_Out Bus Element3/1 -> Out Bus Element3/1
  Bus Selector3/3 -> FAULT_Out Bus Element2/1  "<z>"
  FAULT_Out Bus Element2/1 -> Out Bus Element2/1
  Bus Selector4/3 -> FAULT_Out Bus Element5/1  "<z>"
  FAULT_Out Bus Element5/1 -> Out Bus Element5/1
  Bus Selector5/1 -> FAULT_Out Bus Element6/1  "<altitude>"
  FAULT_Out Bus Element6/1 -> Out Bus Element6/1
  Bus Selector6/1 -> FAULT_Out Bus Element7/1  "<pressure>"
  FAULT_Out Bus Element7/1 -> Out Bus Element7/1
  Bus Selector4/2 -> FAULT_Out Bus Element4/1  "<y>"
  FAULT_Out Bus Element4/1 -> Out Bus Element4/1
  Bus Selector3/1 -> FAULT_Out Bus Element/1  "<x>"
  FAULT_Out Bus Element/1 -> Out Bus Element/1
  Bus Selector3/2 -> FAULT_Out Bus Element1/1  "<y>"
  FAULT_Out Bus Element1/1 -> Out Bus Element1/1
  Bus Selector1/1 -> FAULT_Out Bus Element8/1  "<vbat_V>"
  FAULT_Out Bus Element8/1 -> Out Bus Element8/1
  HAL_vbat_SI/1 -> Bus Selector1/1
  Bus Selector1/2 -> FAULT_Out Bus Element9/1  "<vbat_percentage>"
  FAULT_Out Bus Element9/1 -> Out Bus Element9/1

== system FCS/Crash Predictor Flags/Geofencing error ==
  Action Port : ActionPort
  FAULT_Action Port : F_Line_block/Subsystem
  Constant : Constant  OutDataTypeStr=uint8
  Out1 : Outport
  FAULT_Out1 : F_Line_block/Subsystem
  wires:
  Constant/1 -> FAULT_Out1/1
  FAULT_Out1/1 -> Out1/1

== system FCS/Crash Predictor Flags/Normal condition ==
  Action Port : ActionPort
  FAULT_Action Port : F_Line_block/Subsystem
  Constant : Constant  Value=0  OutDataTypeStr=uint8
  Out1 : Outport
  FAULT_Out1 : F_Line_block/Subsystem
  wires:
  Constant/1 -> FAULT_Out1/1
  FAULT_Out1/1 -> Out1/1

== system FCS/Crash Predictor Flags/estimator/Optical flow error ==
  Action Port : ActionPort
  FAULT_Action Port : F_Line_block/Subsystem
  Constant : Constant  Value=99  OutDataTypeStr=uint8
  Out1 : Outport
  FAULT_Out1 : F_Line_block/Subsystem
  wires:
  Constant/1 -> FAULT_Out1/1
  FAULT_Out1/1 -> Out1/1

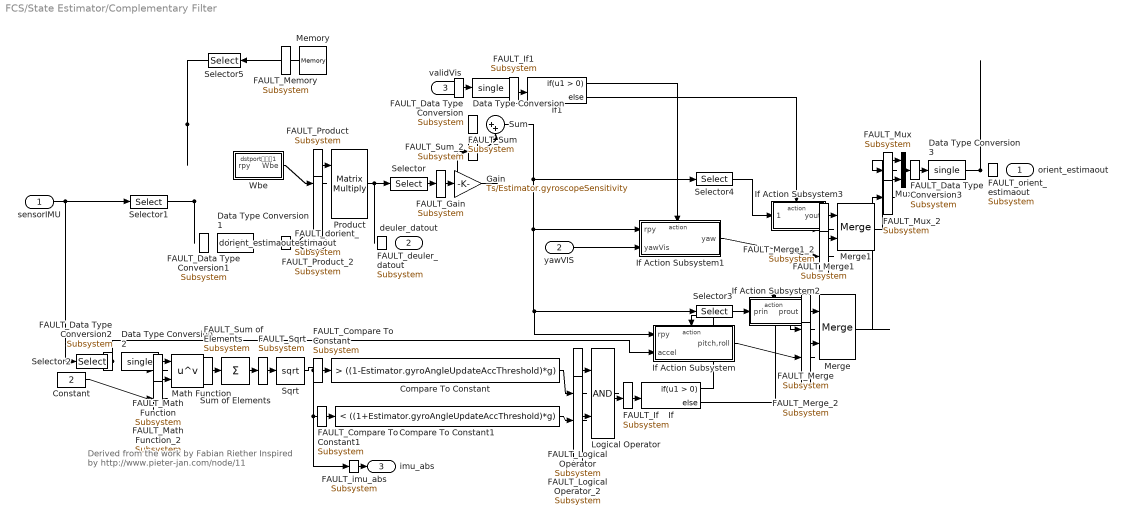
== system FCS/State Estimator/Complementary Filter ==
  note: Derived from the work by Fabian Riether
      | Inspired by http://www.pieter-jan.com/node/11
  sensorIMU : Inport  OutDataTypeStr=single
  yawVIS : Inport  Port=2
  validVis : Inport  Port=3
  Compare To Constant : simulink/Logic and Bit Operations/Compare To Constant  relop=>  const=((1-Estimator.gyroAngleUpdateAccThreshold)*g)  OutDataTypeStr=boolean
  FAULT_Compare To Constant : F_Line_block/Subsystem
  Compare To Constant1 : simulink/Logic and Bit Operations/Compare To Constant  relop=<  const=((1+Estimator.gyroAngleUpdateAccThreshold)*g)  OutDataTypeStr=boolean
  FAULT_Compare To Constant1 : F_Line_block/Subsystem
  Constant : Constant  Value=2  OutDataTypeStr=single
  Data Type Conversion{,1..3} (4 alike) : DataTypeConversion  OutDataTypeStr=single
  FAULT_Data Type Conversion{,1..3} (4 alike) : F_Line_block/Subsystem
  Gain : Gain  Gain=Ts/Estimator.gyroscopeSensitivity
  FAULT_Gain : F_Line_block/Subsystem
  If : If
  FAULT_If : F_Line_block/Subsystem
  If Action Subsystem : Subsystem  TreatAsAtomicUnit=on
  If Action Subsystem1 : Subsystem  TreatAsAtomicUnit=on
  If Action Subsystem2 : Subsystem  TreatAsAtomicUnit=on
  If Action Subsystem3 : Subsystem  TreatAsAtomicUnit=on
  If1 : If
  FAULT_If1 : F_Line_block/Subsystem
  Logical Operator : Logic  AllPortsSameDT=off  OutDataTypeStr=fixdt(1,16)
  FAULT_Logical Operator : F_Line_block/Subsystem
  FAULT_Logical Operator_2 : F_Line_block/Subsystem
  Math Function : Math  Operator=pow  SaturateOnIntegerOverflow=on
  FAULT_Math Function : F_Line_block/Subsystem
  FAULT_Math Function_2 : F_Line_block/Subsystem
  Memory : Memory  InitialCondition=single(Estimator.complementaryFilterInit)  InheritSampleTime=on
  FAULT_Memory : F_Line_block/Subsystem
  Merge : Merge
  FAULT_Merge : F_Line_block/Subsystem
  FAULT_Merge_2 : F_Line_block/Subsystem
  Merge1 : Merge
  FAULT_Merge1 : F_Line_block/Subsystem
  FAULT_Merge1_2 : F_Line_block/Subsystem
  Mux : Mux  Inputs=2
  FAULT_Mux : F_Line_block/Subsystem
  FAULT_Mux_2 : F_Line_block/Subsystem
  Product : Product  Multiplication=Matrix(*)
  FAULT_Product : F_Line_block/Subsystem
  FAULT_Product_2 : F_Line_block/Subsystem
  Selector : Selector  InputPortWidth=3  IndexOptions=Index vector (dialog)  Indices=[3 2 1]  OutputSizes=1
  Selector1 : Selector  InputPortWidth=6  IndexOptions=Index vector (dialog)  Indices=[4 5 6]  OutputSizes=1
  Selector2 : Selector  InputPortWidth=6  IndexOptions=Index vector (dialog)  Indices=[1 2 3]  OutputSizes=1
  Selector3 : Selector  InputPortWidth=3  IndexOptions=Index vector (dialog)  Indices=[2 1]  OutputSizes=1
  Selector4 : Selector  InputPortWidth=3  IndexOptions=Index vector (dialog)  Indices=[3]  OutputSizes=1
  Selector5 : Selector  InputPortWidth=3  IndexOptions=Index vector (dialog)  Indices=[3 2 1]  OutputSizes=1
  Sqrt : Sqrt  SaturateOnIntegerOverflow=on
  FAULT_Sqrt : F_Line_block/Subsystem
  Sum : Sum  Inputs=|++
  FAULT_Sum : F_Line_block/Subsystem
  FAULT_Sum_2 : F_Line_block/Subsystem
  Sum of Elements : Sum  Inputs=+
  FAULT_Sum of Elements : F_Line_block/Subsystem
  Wbe : Subsystem
  orient_estimaout : Outport
  FAULT_orient_estimaout : F_Line_block/Subsystem
  deuler_datout : Outport  Port=2
  FAULT_deuler_datout : F_Line_block/Subsystem
  imu_abs : Outport  Port=3  OutDataTypeStr=single
  FAULT_imu_abs : F_Line_block/Subsystem
  dorient_estimaout : Outport  Port=4
  FAULT_dorient_estimaout : F_Line_block/Subsystem
  wires:
  sensorIMU/1 -> Selector1/1, Selector2/1
  Product/1 -> ?FAULT_deuler_datout_		DstPort			1/1, Selector/1
  ?FAULT_Product3/1 -> ?Product3/1
  ?FAULT_Create 3x3 Matrix/1 -> ?Create 3x3 Matrix/1
  ?FAULT_deuler_datout_		DstPort			1/1 -> deuler_datout/dstport			1
  ?FAULT_Product3_2/1 -> ?Product3/2
  Wbe/1(Wbe) -> FAULT_Product/1
  FAULT_Product/1 -> Product/1
  Selector/1 -> FAULT_Gain/1
  FAULT_Gain/1 -> Gain/1
  Gain/1 -> FAULT_Sum_2/1
  FAULT_Sum_2/1 -> Sum/2
  Memory/1 -> Selector5/1
  Sum of Elements/1 -> FAULT_Sqrt/1
  FAULT_Sqrt/1 -> Sqrt/1
  Math Function/1 -> FAULT_Sum of Elements/1
  FAULT_Sum of Elements/1 -> Sum of Elements/1
  Constant/1 -> FAULT_Math Function_2/1
  FAULT_Math Function_2/1 -> Math Function/2
  Selector2/1 -> If Action Subsystem/2(accel), ?FAULT_Data Type Conversion2_		DstPort			1/1
  ?FAULT_Product3/1 -> ?Product3/1
  ?FAULT_Data Type Conversion2_		DstPort			1/1 -> Data Type Conversion2/dstport			1
  Sqrt/1 -> FAULT_imu_abs/1, Compare To Constant1/1, Compare To Constant/1
  Compare To Constant/1 -> FAULT_Logical Operator/1
  FAULT_Logical Operator/1 -> Logical Operator/1
  Compare To Constant1/1 -> FAULT_Logical Operator_2/1
  FAULT_Logical Operator_2/1 -> Logical Operator/2
  If Action Subsystem/1(pitch,roll) -> FAULT_Merge_2/1
  FAULT_Merge_2/1 -> Merge/2
  Sum/1 -> If Action Subsystem1/1(rpy), If Action Subsystem/1(rpy), Selector3/1, Selector4/1
  Selector3/1 -> If Action Subsystem2/1(prin)
  yawVIS/1 -> If Action Subsystem1/2(yawVis)
  Selector4/1 -> If Action Subsystem3/1(yawin)
  If Action Subsystem1/1(yaw) -> FAULT_Merge1_2/1
  FAULT_imu_abs/1 -> imu_abs/1
  ?FAULT_Data Type Conversion2_		DstPort			1/1 -> Data Type Conversion2/dstport			1
  ?FAULT_deuler_datout_		DstPort			1/1 -> deuler_datout/dstport			1
  ?FAULT_Product3_2/1 -> ?Product3/2
  FAULT_Merge1_2/1 -> Merge1/2
  Merge/1 -> FAULT_Mux_2/1
  FAULT_Mux_2/1 -> Mux/2
  Mux/1 -> FAULT_Data Type Conversion3/1
  FAULT_Data Type Conversion3/1 -> Data Type Conversion3/1
  If Action Subsystem2/1(prout) -> FAULT_Merge/1
  FAULT_Merge/1 -> Merge/1
  If/2 -> If Action Subsystem2/Action
  If Action Subsystem3/1(yout) -> FAULT_Merge1/1
  FAULT_Merge1/1 -> Merge1/1
  If1/2 -> If Action Subsystem3/Action
  Logical Operator/1 -> FAULT_If/1
  FAULT_If/1 -> If/1
  If/1 -> If Action Subsystem/Action
  If1/1 -> If Action Subsystem1/Action
  Data Type Conversion/1 -> FAULT_If1/1
  FAULT_If1/1 -> If1/1
  validVis/1 -> FAULT_Data Type Conversion/1
  FAULT_Data Type Conversion/1 -> Data Type Conversion/1
  Selector1/1 -> ?FAULT_Product_		DstPort			2/1, ?FAULT_Data Type Conversion1_		DstPort			1/1
  ?FAULT_Product_		DstPort			2/1 -> Product/dstport			2
  ?FAULT_Data Type Conversion1_		DstPort			1/1 -> Data Type Conversion1/dstport			1
  Data Type Conversion2/1 -> FAULT_Math Function/1
  FAULT_Math Function/1 -> Math Function/1
  Data Type Conversion3/1 -> ?FAULT_Memory_		DstPort			1/1, ?FAULT_orient_estimaout_		DstPort			1/1
  ?FAULT_Memory_		DstPort			1/1 -> Memory/dstport			1
  ?FAULT_orient_estimaout_		DstPort			1/1 -> orient_estimaout/dstport			1
  Merge1/1 -> FAULT_Mux/1
  FAULT_Mux/1 -> Mux/1
  Selector5/1 -> ?FAULT_Sum_		DstPort			1/1, ?FAULT_Wbe_		DstPort			1/1
  ?FAULT_Sum_		DstPort			1/1 -> Sum/dstport			1
  ?FAULT_Wbe_		DstPort			1/1 -> Wbe/dstport			1
  Data Type Conversion1/1 -> FAULT_dorient_estimaout/1
  FAULT_dorient_estimaout/1 -> dorient_estimaout/1

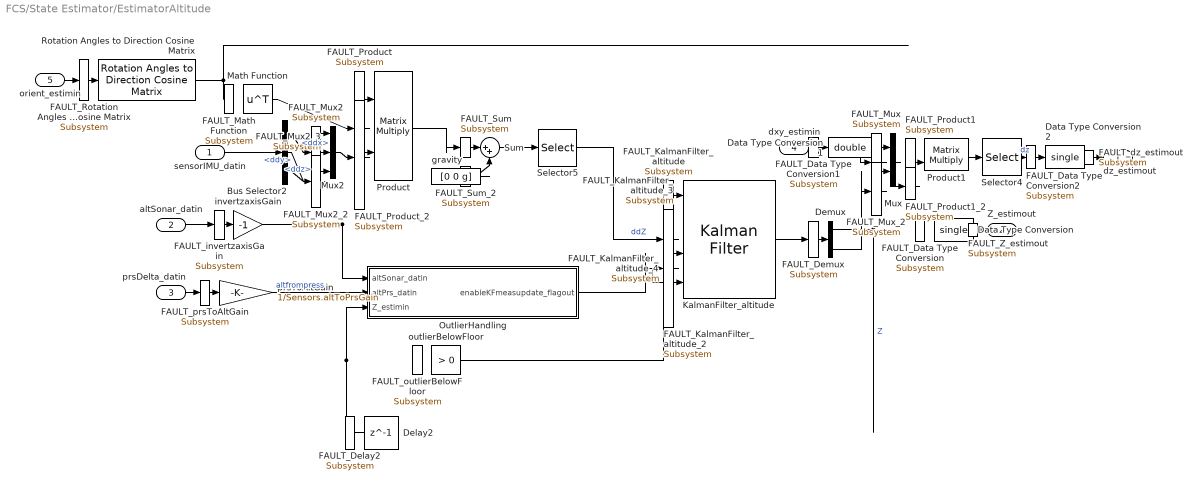
== system FCS/State Estimator/EstimatorAltitude ==
  sensorIMU_datin : Inport
  altSonar_datin : Inport  Port=2
  prsDelta_datin : Inport  Port=3
  dxy_estimin : Inport  Port=4
  orient_estimin : Inport  Port=5
  Bus Selector2 : BusSelector  OutputSignals=ddx,ddy,ddz
  Data Type Conversion : DataTypeConversion  OutDataTypeStr=single  SaturateOnIntegerOverflow=on
  FAULT_Data Type Conversion : F_Line_block/Subsystem
  Data Type Conversion1 : DataTypeConversion  OutDataTypeStr=double  SaturateOnIntegerOverflow=on
  FAULT_Data Type Conversion1 : F_Line_block/Subsystem
  Data Type Conversion2 : DataTypeConversion  OutDataTypeStr=single  SaturateOnIntegerOverflow=on
  FAULT_Data Type Conversion2 : F_Line_block/Subsystem
  Delay2 : Delay  DelayLength=1  InitialCondition=0
  FAULT_Delay2 : F_Line_block/Subsystem
  Demux : Demux  Outputs=2
  FAULT_Demux : F_Line_block/Subsystem
  KalmanFilter_altitude : ctrlSharedLib/Kalman Filter  TimeDomain=Discrete-Time  UseCurrentEstimator=on  ModelSource=Individual A, B, C, D matrices  ModelSourceVariable=sys  A=[1 Ts; 0 1]  B=[0;Ts]  C=[1 0]  D=[0]  NumberOfStates=2  NumberOfInputs=2  NumberOfOutputs=2  InitialEstimateSource=Dialog  X0=[init.posNED(3) 0]  P0=10  UseK=off  UseGH=on  NumberOfProcessNoiseInputs=2  G=Estimator.alt.kf.G  TimeInvariantG=on  H=Estimator.alt.kf.H  TimeInvariantH=on  Q=Estimator.alt.kf.Q  TimeInvariantQ=on  R=Estimator.alt.kf.R  TimeInvariantR=on  N=Estimator.alt.kf.N  TimeInvariantN=on  AddInputPort=on  AddEnablePort=on  ExternalReset=Level hold  OutputEstimatedY=off  OutputP=off  Ts=-1
      settings: SourceProductBaseCode=CT
  FAULT_KalmanFilter_altitude : F_Line_block/Subsystem
  FAULT_KalmanFilter_altitude_2 : F_Line_block/Subsystem
  FAULT_KalmanFilter_altitude_3 : F_Line_block/Subsystem
  FAULT_KalmanFilter_altitude_4 : F_Line_block/Subsystem
  Math Function : Math  Operator=transpose  SaturateOnIntegerOverflow=on
  FAULT_Math Function : F_Line_block/Subsystem
  Mux : Mux  Inputs=2
  FAULT_Mux : F_Line_block/Subsystem
  FAULT_Mux_2 : F_Line_block/Subsystem
  Mux2 : Mux  Inputs=3
  FAULT_Mux2 : F_Line_block/Subsystem
  FAULT_Mux2_2 : F_Line_block/Subsystem
  FAULT_Mux2_3 : F_Line_block/Subsystem
  OutlierHandling : Subsystem
  Product : Product  Multiplication=Matrix(*)
  FAULT_Product : F_Line_block/Subsystem
  FAULT_Product_2 : F_Line_block/Subsystem
  Product1 : Product  Multiplication=Matrix(*)
  FAULT_Product1 : F_Line_block/Subsystem
  FAULT_Product1_2 : F_Line_block/Subsystem
  Rotation Angles to Direction Cosine Matrix : sharedtransform/Rotation Angles to Direction Cosine Matrix  rotationOrder=ZYX  aMode=aMode
      settings: SourceProductBaseCode=AE
  FAULT_Rotation Angles to Direction Cosine Matrix : F_Line_block/Subsystem
  Selector4 : Selector  InputPortWidth=3  IndexOptions=Index vector (dialog)  Indices=[3]  OutputSizes=1
  Selector5 : Selector  InputPortWidth=3  IndexOptions=Index vector (dialog)  Indices=[3]  OutputSizes=1
  Sum : Sum  Inputs=|++
  FAULT_Sum : F_Line_block/Subsystem
  FAULT_Sum_2 : F_Line_block/Subsystem
  gravity : Constant  Value=[0 0 g]
  invertzaxisGain : Gain  Gain=-1  ParamDataTypeStr=single  OutDataTypeStr=double
  FAULT_invertzaxisGain : F_Line_block/Subsystem
  outlierBelowFloor : simulink/Logic and Bit Operations/Compare To Constant  relop=>  const=0  OutDataTypeStr=boolean
  FAULT_outlierBelowFloor : F_Line_block/Subsystem
  prsToAltGain : Gain  Gain=1/Sensors.altToPrsGain
  FAULT_prsToAltGain : F_Line_block/Subsystem
  dz_estimout : Outport
  FAULT_dz_estimout : F_Line_block/Subsystem
  Z_estimout : Outport  Port=2
  FAULT_Z_estimout : F_Line_block/Subsystem
  wires:
  Mux2/1 -> FAULT_Product_2/1
  FAULT_Product_2/1 -> Product/2
  sensorIMU_datin/1 -> Bus Selector2/1
  Bus Selector2/3 -> FAULT_Mux2_3/1  "<ddz>"
  FAULT_Mux2_3/1 -> Mux2/3
  Bus Selector2/2 -> FAULT_Mux2_2/1  "<ddy>"
  FAULT_Mux2_2/1 -> Mux2/2
  Bus Selector2/1 -> FAULT_Mux2/1  "<ddx>"
  FAULT_Mux2/1 -> Mux2/1
  Product1/1 -> Selector4/1
  dxy_estimin/1 -> FAULT_Data Type Conversion1/1
  FAULT_Data Type Conversion1/1 -> Data Type Conversion1/1
  Delay2/1 -> OutlierHandling/3(Z_estimin), ?FAULT_outlierBelowFloor_		DstPort			1/1
  ?FAULT_Add1/1 -> ?Add1/1
  ?FAULT_outlierBelowFloor_		DstPort			1/1 -> outlierBelowFloor/dstport			1
  prsToAltGain/1 -> OutlierHandling/2(altPrs_datin)  "altfrompress"
  prsDelta_datin/1 -> FAULT_prsToAltGain/1
  FAULT_prsToAltGain/1 -> prsToAltGain/1
  outlierBelowFloor/1 -> FAULT_KalmanFilter_altitude_4/1
  FAULT_KalmanFilter_altitude_4/1 -> KalmanFilter_altitude/4
  Demux/2 -> FAULT_Mux_2/1
  FAULT_Mux_2/1 -> Mux/2
  Selector4/1 -> FAULT_Data Type Conversion2/1  "dz"
  FAULT_Data Type Conversion2/1 -> Data Type Conversion2/1
  Demux/1 -> ?FAULT_Data Type Conversion_		DstPort			1/1, ?FAULT_Delay2_		DstPort			1/1  "Z"
  ?FAULT_Data Type Conversion_		DstPort			1/1 -> Data Type Conversion/dstport			1
  ?FAULT_Delay2_		DstPort			1/1 -> Delay2/dstport			1
  Selector5/1 -> FAULT_KalmanFilter_altitude/1  "ddZ"
  FAULT_KalmanFilter_altitude/1 -> KalmanFilter_altitude/1
  Mux/1 -> FAULT_Product1_2/1
  FAULT_Product1_2/1 -> Product1/2
  KalmanFilter_altitude/1 -> FAULT_Demux/1
  FAULT_Demux/1 -> Demux/1
  Sum/1 -> Selector5/1
  gravity/1 -> FAULT_Sum_2/1
  FAULT_Sum_2/1 -> Sum/2
  Product/1 -> FAULT_Sum/1
  FAULT_Sum/1 -> Sum/1
  altSonar_datin/1 -> FAULT_invertzaxisGain/1
  FAULT_invertzaxisGain/1 -> invertzaxisGain/1
  orient_estimin/1 -> FAULT_Rotation Angles to Direction Cosine Matrix/1
  FAULT_Rotation Angles to Direction Cosine Matrix/1 -> Rotation Angles to Direction Cosine Matrix/1
  Data Type Conversion/1 -> FAULT_Z_estimout/1
  FAULT_Z_estimout/1 -> Z_estimout/1
  Data Type Conversion1/1 -> FAULT_Mux/1
  FAULT_Mux/1 -> Mux/1
  Math Function/1 -> FAULT_Product/1
  FAULT_Product/1 -> Product/1
  invertzaxisGain/1 -> ?FAULT_KalmanFilter_altitude_		DstPort			2/1, OutlierHandling/1(altSonar_datin)
  ?FAULT_KalmanFilter_altitude_		DstPort			2/1 -> KalmanFilter_altitude/dstport			2
  ?FAULT_Delay2_		DstPort			1/1 -> Delay2/dstport			1
  Data Type Conversion2/1 -> FAULT_dz_estimout/1
  FAULT_dz_estimout/1 -> dz_estimout/1
  OutlierHandling/1(enableKFmeasupdate_flagout) -> FAULT_KalmanFilter_altitude_3/1
  FAULT_KalmanFilter_altitude_3/1 -> KalmanFilter_altitude/3
  Rotation Angles to Direction Cosine Matrix/1 -> ?FAULT_Math Function_		DstPort			1/1, ?FAULT_Product1_		DstPort			1/1
  ?FAULT_Math Function_		DstPort			1/1 -> Math Function/dstport			1
  ?FAULT_Product1_		DstPort			1/1 -> Product1/dstport			1

== system FCS/State Estimator/EstimatorXYPosition ==
  opticalFlow_datin : Inport
  controlModePosVSOrient_flagin : Inport  Port=2
  usePosVIS_flagin : Inport  Port=3
  posVIS_datin : Inport  Port=4
  sensorIMU_datin : Inport  Port=5
  Z_estimin : Inport  Port=6
  dz_estimin : Inport  Port=7
  orient_estimin : Inport  Port=8
  EstimatorVelocity : Subsystem
  EstimatorXYPosition : Subsystem
  XY_estimout : Outport
  FAULT_XY_estimout : F_Line_block/Subsystem
  dxy_estimout : Outport  Port=2
  FAULT_dxy_estimout : F_Line_block/Subsystem
  wires:
  EstimatorXYPosition/1(XY_estimout) -> FAULT_XY_estimout/1
  FAULT_XY_estimout/1 -> XY_estimout/1
  usePosVIS_flagin/1 -> EstimatorXYPosition/6(usePosVIS_flagin)
  posVIS_datin/1 -> EstimatorXYPosition/5(posVIS_datin)
  dz_estimin/1 -> EstimatorXYPosition/4(dz_estimin)
  controlModePosVSOrient_flagin/1 -> EstimatorXYPosition/3(controlModePosVSOrient_flagin)
  Z_estimin/1 -> EstimatorVelocity/2(Z_estimin)
  sensorIMU_datin/1 -> EstimatorVelocity/3(sensorIMU_datin)
  opticalFlow_datin/1 -> EstimatorVelocity/1(opticalFlow_datin)
  EstimatorVelocity/1(dxy_estimout) -> ?FAULT_dxy_estimout_		DstPort			1/1, EstimatorXYPosition/1(dxy_estimin)
  ?FAULT_dxy_estimout_		DstPort			1/1 -> dxy_estimout/dstport			1
  ?FAULT_KalmanFilter_posxy/1 -> ?KalmanFilter_posxy/1
  orient_estimin/1 -> EstimatorXYPosition/2(orient_estimin), EstimatorVelocity/4(orient_estimin)
